simulink model "model1"  (R2017a)
settings: Solver=VariableStepAuto  StartTime=0.0  StopTime=10  RelTol=1e-3
values from neighbouring files (symbols this model uses):
  R = r0*[1 -1]    [Param.m]
  S = [s1 s0]    [Param.m]
  T = [s1 s0]    [Param.m]
  Te = 1e-3    (= 0.001)    [Param.m]
settings Model: Creator=arek  LastModifiedBy=GANOU Arouna

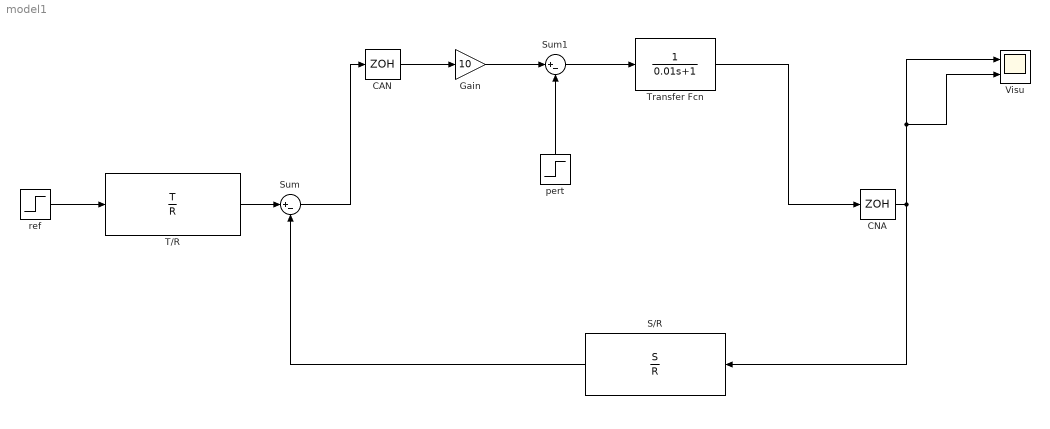
== system model1 ==
  CAN : ZeroOrderHold  SampleTime=-1
  CNA : ZeroOrderHold  SampleTime=-1
  Gain : Gain  Gain=10
  S/R : DiscreteTransferFcn  Numerator=S  Denominator=R  SampleTime=Te
  Sum : Sum  Inputs=|+-
  Sum1 : Sum  Inputs=|+-
  T/R : DiscreteTransferFcn  Numerator=T  Denominator=R  SampleTime=Te
  Transfer Fcn : TransferFcn  Denominator=[0.01 1]
  Visu : Scope  NumInputPorts=2
  pert : Step  Time=5  SampleTime=Te
  ref : Step  Time=0  SampleTime=Te
  wires:
  S/R/1 -> Sum/2
  T/R/1 -> Sum/1
  Transfer Fcn/1 -> CNA/1
  CNA/1 -> Visu/2, Visu/1, S/R/1
  ref/1 -> T/R/1
  Sum/1 -> CAN/1
  CAN/1 -> Gain/1
  Gain/1 -> Sum1/1
  Sum1/1 -> Transfer Fcn/1
  pert/1 -> Sum1/2
